simulink model "speed_pi_compare_tb"  (R2026b)
settings: Solver=FixedStepDiscrete  StopTime=0.01  FixedStep=0.0001
model workspace (MAT data in the model file):
  Iq_int_limit = 0.5
  Kaw_s = 0.08
  Ki_ASR = 1.44267798821
  Kp_ASR = 0.0180334748527
  Speed_loop_Iq_Limit = 1
  Ts = 0.0001
  Ts_ASR = 0.001
  v_ff_eps = 0.5
  v_over_eps = 3
  v_ref_zero_eps = 0
undefined symbols (not defined in the file): Iq_fric_run, Iq_fric_start, v_stick_off, v_stick_on
libraries: simulink x7

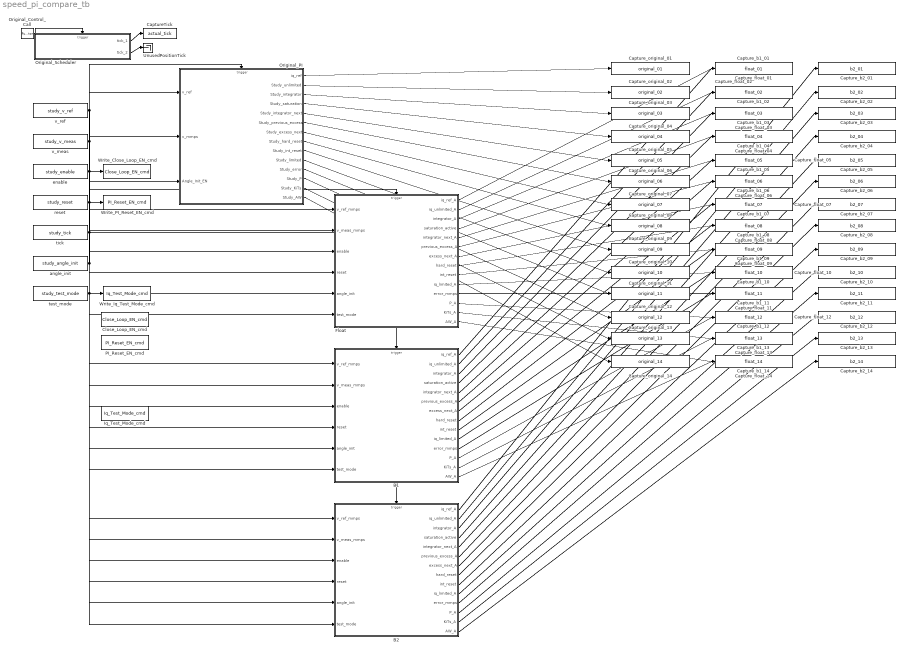
== system speed_pi_compare_tb ==
  B1 : Subsystem
  B2 : Subsystem
  CaptureTick : ToWorkspace  VariableName=actual_tick  SaveFormat=Timeseries
  Capture_b1_01 : ToWorkspace  VariableName=b1_01  SaveFormat=Timeseries
  Capture_b1_02 : ToWorkspace  VariableName=b1_02  SaveFormat=Timeseries
  Capture_b1_03 : ToWorkspace  VariableName=b1_03  SaveFormat=Timeseries
  Capture_b1_04 : ToWorkspace  VariableName=b1_04  SaveFormat=Timeseries
  Capture_b1_05 : ToWorkspace  VariableName=b1_05  SaveFormat=Timeseries
  Capture_b1_06 : ToWorkspace  VariableName=b1_06  SaveFormat=Timeseries
  Capture_b1_07 : ToWorkspace  VariableName=b1_07  SaveFormat=Timeseries
  Capture_b1_08 : ToWorkspace  VariableName=b1_08  SaveFormat=Timeseries
  Capture_b1_09 : ToWorkspace  VariableName=b1_09  SaveFormat=Timeseries
  Capture_b1_10 : ToWorkspace  VariableName=b1_10  SaveFormat=Timeseries
  Capture_b1_11 : ToWorkspace  VariableName=b1_11  SaveFormat=Timeseries
  Capture_b1_12 : ToWorkspace  VariableName=b1_12  SaveFormat=Timeseries
  Capture_b1_13 : ToWorkspace  VariableName=b1_13  SaveFormat=Timeseries
  Capture_b1_14 : ToWorkspace  VariableName=b1_14  SaveFormat=Timeseries
  Capture_b2_01 : ToWorkspace  VariableName=b2_01  SaveFormat=Timeseries
  Capture_b2_02 : ToWorkspace  VariableName=b2_02  SaveFormat=Timeseries
  Capture_b2_03 : ToWorkspace  VariableName=b2_03  SaveFormat=Timeseries
  Capture_b2_04 : ToWorkspace  VariableName=b2_04  SaveFormat=Timeseries
  Capture_b2_05 : ToWorkspace  VariableName=b2_05  SaveFormat=Timeseries
  Capture_b2_06 : ToWorkspace  VariableName=b2_06  SaveFormat=Timeseries
  Capture_b2_07 : ToWorkspace  VariableName=b2_07  SaveFormat=Timeseries
  Capture_b2_08 : ToWorkspace  VariableName=b2_08  SaveFormat=Timeseries
  Capture_b2_09 : ToWorkspace  VariableName=b2_09  SaveFormat=Timeseries
  Capture_b2_10 : ToWorkspace  VariableName=b2_10  SaveFormat=Timeseries
  Capture_b2_11 : ToWorkspace  VariableName=b2_11  SaveFormat=Timeseries
  Capture_b2_12 : ToWorkspace  VariableName=b2_12  SaveFormat=Timeseries
  Capture_b2_13 : ToWorkspace  VariableName=b2_13  SaveFormat=Timeseries
  Capture_b2_14 : ToWorkspace  VariableName=b2_14  SaveFormat=Timeseries
  Capture_float_01 : ToWorkspace  VariableName=float_01  SaveFormat=Timeseries
  Capture_float_02 : ToWorkspace  VariableName=float_02  SaveFormat=Timeseries
  Capture_float_03 : ToWorkspace  VariableName=float_03  SaveFormat=Timeseries
  Capture_float_04 : ToWorkspace  VariableName=float_04  SaveFormat=Timeseries
  Capture_float_05 : ToWorkspace  VariableName=float_05  SaveFormat=Timeseries
  Capture_float_06 : ToWorkspace  VariableName=float_06  SaveFormat=Timeseries
  Capture_float_07 : ToWorkspace  VariableName=float_07  SaveFormat=Timeseries
  Capture_float_08 : ToWorkspace  VariableName=float_08  SaveFormat=Timeseries
  Capture_float_09 : ToWorkspace  VariableName=float_09  SaveFormat=Timeseries
  Capture_float_10 : ToWorkspace  VariableName=float_10  SaveFormat=Timeseries
  Capture_float_11 : ToWorkspace  VariableName=float_11  SaveFormat=Timeseries
  Capture_float_12 : ToWorkspace  VariableName=float_12  SaveFormat=Timeseries
  Capture_float_13 : ToWorkspace  VariableName=float_13  SaveFormat=Timeseries
  Capture_float_14 : ToWorkspace  VariableName=float_14  SaveFormat=Timeseries
  Capture_original_01 : ToWorkspace  VariableName=original_01  SaveFormat=Timeseries
  Capture_original_02 : ToWorkspace  VariableName=original_02  SaveFormat=Timeseries
  Capture_original_03 : ToWorkspace  VariableName=original_03  SaveFormat=Timeseries
  Capture_original_04 : ToWorkspace  VariableName=original_04  SaveFormat=Timeseries
  Capture_original_05 : ToWorkspace  VariableName=original_05  SaveFormat=Timeseries
  Capture_original_06 : ToWorkspace  VariableName=original_06  SaveFormat=Timeseries
  Capture_original_07 : ToWorkspace  VariableName=original_07  SaveFormat=Timeseries
  Capture_original_08 : ToWorkspace  VariableName=original_08  SaveFormat=Timeseries
  Capture_original_09 : ToWorkspace  VariableName=original_09  SaveFormat=Timeseries
  Capture_original_10 : ToWorkspace  VariableName=original_10  SaveFormat=Timeseries
  Capture_original_11 : ToWorkspace  VariableName=original_11  SaveFormat=Timeseries
  Capture_original_12 : ToWorkspace  VariableName=original_12  SaveFormat=Timeseries
  Capture_original_13 : ToWorkspace  VariableName=original_13  SaveFormat=Timeseries
  Capture_original_14 : ToWorkspace  VariableName=original_14  SaveFormat=Timeseries
  Close_Loop_EN_cmd : DataStoreMemory  DataStoreName=Close_Loop_EN_cmd  ShowAdditionalParam=off
  Float : Subsystem
  Iq_Test_Mode_cmd : DataStoreMemory  DataStoreName=Iq_Test_Mode_cmd  ShowAdditionalParam=off
  Original_Control_Call : FunctionCallGenerator  SampleTime=Ts
  Original_PI : Subsystem  TreatAsAtomicUnit=on
  Original_Scheduler : Subsystem
  PI_Reset_EN_cmd : DataStoreMemory  DataStoreName=PI_Reset_EN_cmd  ShowAdditionalParam=off
  UnusedPositionTick : Terminator
  Write_Close_Loop_EN_cmd : DataStoreWrite  Priority=-10  DataStoreName=Close_Loop_EN_cmd  IndexOptions=Index vector (dialog)  Indices=1  OutputSizes=1
  Write_Iq_Test_Mode_cmd : DataStoreWrite  Priority=-10  DataStoreName=Iq_Test_Mode_cmd  IndexOptions=Index vector (dialog)  Indices=1  OutputSizes=1
  Write_PI_Reset_EN_cmd : DataStoreWrite  Priority=-10  DataStoreName=PI_Reset_EN_cmd  IndexOptions=Index vector (dialog)  Indices=1  OutputSizes=1
  angle_init : FromWorkspace  VariableName=study_angle_init  SampleTime=0.0001  Interpolate=off  OutputAfterFinalValue=Holding final value
  enable : FromWorkspace  VariableName=study_enable  SampleTime=0.0001  Interpolate=off  OutputAfterFinalValue=Holding final value
  reset : FromWorkspace  VariableName=study_reset  SampleTime=0.0001  Interpolate=off  OutputAfterFinalValue=Holding final value
  test_mode : FromWorkspace  VariableName=study_test_mode  SampleTime=0.0001  Interpolate=off  OutputAfterFinalValue=Holding final value
  tick : FromWorkspace  VariableName=study_tick  SampleTime=0.0001  Interpolate=off  OutputAfterFinalValue=Holding final value
  v_meas : FromWorkspace  VariableName=study_v_meas  SampleTime=0.0001  Interpolate=off  OutputAfterFinalValue=Holding final value
  v_ref : FromWorkspace  VariableName=study_v_ref  SampleTime=0.0001  Interpolate=off  OutputAfterFinalValue=Holding final value
  wires:
  Original_Control_Call/1 -> Original_Scheduler/Trigger
  Original_Scheduler/2(tick_2) -> UnusedPositionTick/1
  Original_Scheduler/1(tick_1) -> CaptureTick/1
  v_ref/1 -> Original_PI/1(v_ref), Float/1(v_ref_mmps), B1/1(v_ref_mmps), B2/1(v_ref_mmps)
  v_meas/1 -> Original_PI/2(v_mmps), Float/2(v_meas_mmps), B1/2(v_meas_mmps), B2/2(v_meas_mmps)
  angle_init/1 -> Original_PI/3(Angle_Init_EN), Float/5(angle_init), B1/5(angle_init), B2/5(angle_init)
  tick/1 -> Original_PI/Trigger, Float/Trigger, B1/Trigger, B2/Trigger
  enable/1 -> Write_Close_Loop_EN_cmd/1, Float/3(enable), B1/3(enable), B2/3(enable)
  reset/1 -> Write_PI_Reset_EN_cmd/1, Float/4(reset), B1/4(reset), B2/4(reset)
  test_mode/1 -> Write_Iq_Test_Mode_cmd/1, Float/6(test_mode), B1/6(test_mode), B2/6(test_mode)
  Original_PI/1(iq_ref) -> Capture_original_01/1
  Original_PI/2(Study_unlimited) -> Capture_original_02/1
  Original_PI/3(Study_integrator) -> Capture_original_03/1
  Original_PI/4(Study_saturation) -> Capture_original_04/1
  Original_PI/5(Study_integrator_next) -> Capture_original_05/1
  Original_PI/6(Study_previous_excess) -> Capture_original_06/1
  Original_PI/7(Study_excess_next) -> Capture_original_07/1
  Original_PI/8(Study_hard_reset) -> Capture_original_08/1
  Original_PI/9(Study_int_reset) -> Capture_original_09/1
  Original_PI/10(Study_limited) -> Capture_original_10/1
  Original_PI/11(Study_error) -> Capture_original_11/1
  Original_PI/12(Study_P) -> Capture_original_12/1
  Original_PI/13(Study_KiTs) -> Capture_original_13/1
  Original_PI/14(Study_AW) -> Capture_original_14/1
  Float/1(iq_ref_A) -> Capture_float_01/1
  Float/2(iq_unlimited_A) -> Capture_float_02/1
  Float/3(integrator_A) -> Capture_float_03/1
  Float/4(saturation_active) -> Capture_float_04/1
  Float/5(integrator_next_A) -> Capture_float_05/1
  Float/6(previous_excess_A) -> Capture_float_06/1
  Float/7(excess_next_A) -> Capture_float_07/1
  Float/8(hard_reset) -> Capture_float_08/1
  Float/9(int_reset) -> Capture_float_09/1
  Float/10(iq_limited_A) -> Capture_float_10/1
  Float/11(error_mmps) -> Capture_float_11/1
  Float/12(P_A) -> Capture_float_12/1
  Float/13(KiTs_A) -> Capture_float_13/1
  Float/14(AW_A) -> Capture_float_14/1
  B1/1(iq_ref_A) -> Capture_b1_01/1
  B1/2(iq_unlimited_A) -> Capture_b1_02/1
  B1/3(integrator_A) -> Capture_b1_03/1
  B1/4(saturation_active) -> Capture_b1_04/1
  B1/5(integrator_next_A) -> Capture_b1_05/1
  B1/6(previous_excess_A) -> Capture_b1_06/1
  B1/7(excess_next_A) -> Capture_b1_07/1
  B1/8(hard_reset) -> Capture_b1_08/1
  B1/9(int_reset) -> Capture_b1_09/1
  B1/10(iq_limited_A) -> Capture_b1_10/1
  B1/11(error_mmps) -> Capture_b1_11/1
  B1/12(P_A) -> Capture_b1_12/1
  B1/13(KiTs_A) -> Capture_b1_13/1
  B1/14(AW_A) -> Capture_b1_14/1
  B2/1(iq_ref_A) -> Capture_b2_01/1
  B2/2(iq_unlimited_A) -> Capture_b2_02/1
  B2/3(integrator_A) -> Capture_b2_03/1
  B2/4(saturation_active) -> Capture_b2_04/1
  B2/5(integrator_next_A) -> Capture_b2_05/1
  B2/6(previous_excess_A) -> Capture_b2_06/1
  B2/7(excess_next_A) -> Capture_b2_07/1
  B2/8(hard_reset) -> Capture_b2_08/1
  B2/9(int_reset) -> Capture_b2_09/1
  B2/10(iq_limited_A) -> Capture_b2_10/1
  B2/11(error_mmps) -> Capture_b2_11/1
  B2/12(P_A) -> Capture_b2_12/1
  B2/13(KiTs_A) -> Capture_b2_13/1
  B2/14(AW_A) -> Capture_b2_14/1

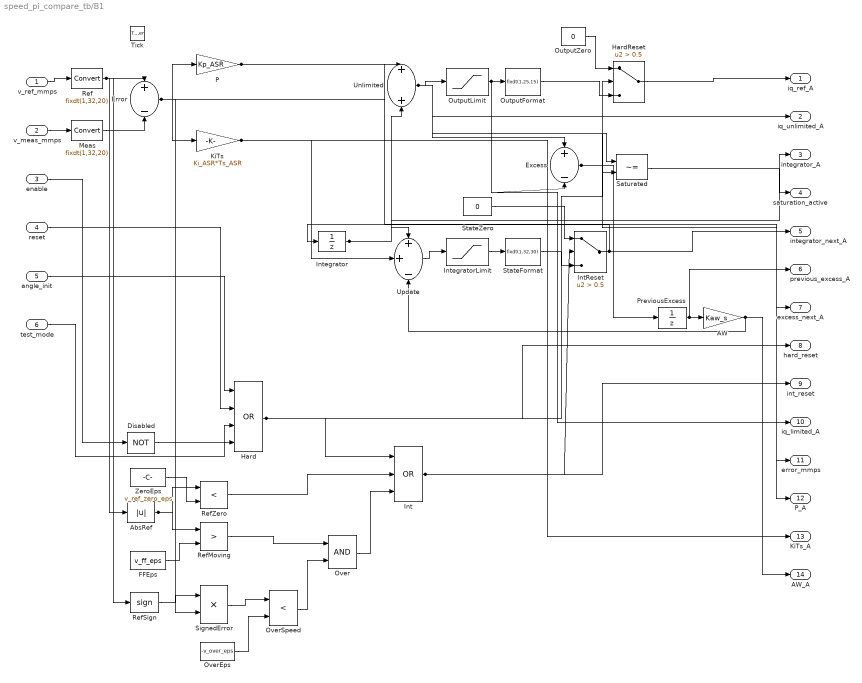
== system speed_pi_compare_tb/B1 ==
  v_ref_mmps : Inport
  v_meas_mmps : Inport  Port=2
  enable : Inport  Port=3
  reset : Inport  Port=4
  angle_init : Inport  Port=5
  test_mode : Inport  Port=6
  Tick : TriggerPort  VariantControl=(inherit)
  AW : Gain  Gain=Kaw_s  ParamDataTypeStr=fixdt(0,32,30)  OutDataTypeStr=fixdt(1,40,30)  RndMeth=Convergent  SaturateOnIntegerOverflow=on
  AbsRef : Abs  RndMeth=Convergent
  Disabled : Logic  Operator=NOT  AllPortsSameDT=off  OutDataTypeStr=boolean
  Error : Sum  Inputs=+-  OutDataTypeStr=fixdt(1,33,20)  AccumDataTypeStr=fixdt(1,33,20)  RndMeth=Convergent  SaturateOnIntegerOverflow=on
  Excess : Sum  Inputs=+-  OutDataTypeStr=fixdt(1,40,30)  AccumDataTypeStr=fixdt(1,44,30)  RndMeth=Convergent  SaturateOnIntegerOverflow=on
  FFEps : Constant  Value=v_ff_eps  OutDataTypeStr=fixdt(1,32,20)
  Hard : Logic  Operator=OR  Inputs=4  AllPortsSameDT=off  OutDataTypeStr=boolean
  HardReset : Switch  Criteria=u2 > Threshold  Threshold=0.5  RndMeth=Convergent  InputSameDT=off
  Int : Logic  Operator=OR  Inputs=3  AllPortsSameDT=off  OutDataTypeStr=boolean
  IntReset : Switch  Criteria=u2 > Threshold  Threshold=0.5  RndMeth=Convergent  InputSameDT=off
  Integrator : UnitDelay  SampleTime=-1
  IntegratorLimit : Saturate  UpperLimit=Iq_int_limit  LowerLimit=-Iq_int_limit  RndMeth=Convergent
  KiTs : Gain  Gain=Ki_ASR*Ts_ASR  ParamDataTypeStr=fixdt(0,32,30)  OutDataTypeStr=fixdt(1,40,30)  RndMeth=Convergent  SaturateOnIntegerOverflow=on
  Meas : DataTypeConversion  OutDataTypeStr=fixdt(1,32,20)  RndMeth=Convergent
  OutputFormat : DataTypeConversion  OutDataTypeStr=fixdt(1,25,15)  RndMeth=Convergent
  OutputLimit : Saturate  UpperLimit=Speed_loop_Iq_Limit  LowerLimit=-Speed_loop_Iq_Limit  RndMeth=Convergent
  OutputZero : Constant  Value=0  OutDataTypeStr=fixdt(1,25,15)
  Over : Logic  AllPortsSameDT=off  OutDataTypeStr=boolean
  OverEps : Constant  Value=-v_over_eps  OutDataTypeStr=fixdt(1,33,20)
  OverSpeed : RelationalOperator  Operator=<  RndMeth=Convergent  InputSameDT=off
  P : Gain  Gain=Kp_ASR  ParamDataTypeStr=fixdt(0,32,30)  OutDataTypeStr=fixdt(1,40,30)  RndMeth=Convergent  SaturateOnIntegerOverflow=on
  PreviousExcess : UnitDelay  SampleTime=-1
  Ref : DataTypeConversion  OutDataTypeStr=fixdt(1,32,20)  RndMeth=Convergent
  RefMoving : RelationalOperator  Operator=>  RndMeth=Convergent  InputSameDT=off
  RefSign : Signum
  RefZero : RelationalOperator  Operator=<  RndMeth=Convergent  InputSameDT=off
  Saturated : RelationalOperator  Operator=~=  RndMeth=Convergent  InputSameDT=off
  SignedError : Product  OutDataTypeStr=fixdt(1,33,20)  RndMeth=Convergent  SaturateOnIntegerOverflow=on
  StateFormat : DataTypeConversion  OutDataTypeStr=fixdt(1,32,30)  RndMeth=Convergent
  StateZero : Constant  Value=0  OutDataTypeStr=fixdt(1,32,30)
  Unlimited : Sum  OutDataTypeStr=fixdt(1,42,30)  AccumDataTypeStr=fixdt(1,44,30)  RndMeth=Convergent  SaturateOnIntegerOverflow=on
  Update : Sum  Inputs=++-  OutDataTypeStr=fixdt(1,44,30)  AccumDataTypeStr=fixdt(1,44,30)  RndMeth=Convergent  SaturateOnIntegerOverflow=on
  ZeroEps : Constant  Value=v_ref_zero_eps  OutDataTypeStr=fixdt(1,32,20)
  iq_ref_A : Outport
  iq_unlimited_A : Outport  Port=2
  integrator_A : Outport  Port=3
  saturation_active : Outport  Port=4
  integrator_next_A : Outport  Port=5
  previous_excess_A : Outport  Port=6
  excess_next_A : Outport  Port=7
  hard_reset : Outport  Port=8
  int_reset : Outport  Port=9
  iq_limited_A : Outport  Port=10
  error_mmps : Outport  Port=11
  P_A : Outport  Port=12
  KiTs_A : Outport  Port=13
  AW_A : Outport  Port=14
  wires:
  Saturated/1 -> saturation_active/1
  HardReset/1 -> iq_ref_A/1
  Over/1 -> Int/3
  RefZero/1 -> Int/2
  OverSpeed/1 -> Over/2
  RefMoving/1 -> Over/1
  OverEps/1 -> OverSpeed/2
  SignedError/1 -> OverSpeed/1
  RefSign/1 -> SignedError/1
  FFEps/1 -> RefMoving/2
  ZeroEps/1 -> RefZero/2
  AbsRef/1 -> RefMoving/1, RefZero/1
  Disabled/1 -> Hard/4
  test_mode/1 -> Hard/3
  reset/1 -> Hard/2
  angle_init/1 -> Hard/1
  enable/1 -> Disabled/1
  OutputFormat/1 -> HardReset/3
  Hard/1 -> hard_reset/1, Int/1, HardReset/2
  OutputZero/1 -> HardReset/1
  IntReset/1 -> integrator_next_A/1, Integrator/1
  StateFormat/1 -> IntReset/3
  Int/1 -> int_reset/1, IntReset/2
  StateZero/1 -> IntReset/1
  IntegratorLimit/1 -> StateFormat/1
  Update/1 -> IntegratorLimit/1
  AW/1 -> AW_A/1, Update/3
  KiTs/1 -> KiTs_A/1, Update/2
  PreviousExcess/1 -> previous_excess_A/1, AW/1
  Excess/1 -> excess_next_A/1, PreviousExcess/1
  OutputLimit/1 -> iq_limited_A/1, Saturated/2, Excess/2, OutputFormat/1
  Unlimited/1 -> iq_unlimited_A/1, Saturated/1, Excess/1, OutputLimit/1
  Integrator/1 -> integrator_A/1, Update/1, Unlimited/2
  P/1 -> P_A/1, Unlimited/1
  Error/1 -> error_mmps/1, SignedError/2, KiTs/1, P/1
  Meas/1 -> Error/2
  Ref/1 -> RefSign/1, AbsRef/1, Error/1
  v_meas_mmps/1 -> Meas/1
  v_ref_mmps/1 -> Ref/1

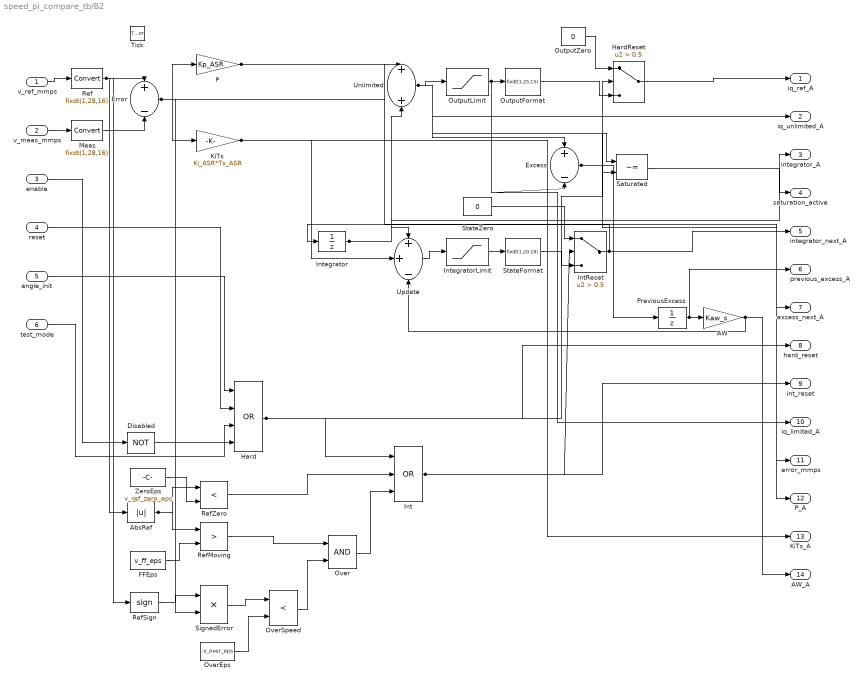
== system speed_pi_compare_tb/B2 ==
  v_ref_mmps : Inport
  v_meas_mmps : Inport  Port=2
  enable : Inport  Port=3
  reset : Inport  Port=4
  angle_init : Inport  Port=5
  test_mode : Inport  Port=6
  Tick : TriggerPort  VariantControl=(inherit)
  AW : Gain  Gain=Kaw_s  ParamDataTypeStr=fixdt(0,24,22)  OutDataTypeStr=fixdt(1,28,18)  RndMeth=Convergent  SaturateOnIntegerOverflow=on
  AbsRef : Abs  RndMeth=Convergent
  Disabled : Logic  Operator=NOT  AllPortsSameDT=off  OutDataTypeStr=boolean
  Error : Sum  Inputs=+-  OutDataTypeStr=fixdt(1,29,16)  AccumDataTypeStr=fixdt(1,29,16)  RndMeth=Convergent  SaturateOnIntegerOverflow=on
  Excess : Sum  Inputs=+-  OutDataTypeStr=fixdt(1,28,18)  AccumDataTypeStr=fixdt(1,32,18)  RndMeth=Convergent  SaturateOnIntegerOverflow=on
  FFEps : Constant  Value=v_ff_eps  OutDataTypeStr=fixdt(1,28,16)
  Hard : Logic  Operator=OR  Inputs=4  AllPortsSameDT=off  OutDataTypeStr=boolean
  HardReset : Switch  Criteria=u2 > Threshold  Threshold=0.5  RndMeth=Convergent  InputSameDT=off
  Int : Logic  Operator=OR  Inputs=3  AllPortsSameDT=off  OutDataTypeStr=boolean
  IntReset : Switch  Criteria=u2 > Threshold  Threshold=0.5  RndMeth=Convergent  InputSameDT=off
  Integrator : UnitDelay  SampleTime=-1
  IntegratorLimit : Saturate  UpperLimit=Iq_int_limit  LowerLimit=-Iq_int_limit  RndMeth=Convergent
  KiTs : Gain  Gain=Ki_ASR*Ts_ASR  ParamDataTypeStr=fixdt(0,24,22)  OutDataTypeStr=fixdt(1,28,18)  RndMeth=Convergent  SaturateOnIntegerOverflow=on
  Meas : DataTypeConversion  OutDataTypeStr=fixdt(1,28,16)  RndMeth=Convergent
  OutputFormat : DataTypeConversion  OutDataTypeStr=fixdt(1,25,15)  RndMeth=Convergent
  OutputLimit : Saturate  UpperLimit=Speed_loop_Iq_Limit  LowerLimit=-Speed_loop_Iq_Limit  RndMeth=Convergent
  OutputZero : Constant  Value=0  OutDataTypeStr=fixdt(1,25,15)
  Over : Logic  AllPortsSameDT=off  OutDataTypeStr=boolean
  OverEps : Constant  Value=-v_over_eps  OutDataTypeStr=fixdt(1,29,16)
  OverSpeed : RelationalOperator  Operator=<  RndMeth=Convergent  InputSameDT=off
  P : Gain  Gain=Kp_ASR  ParamDataTypeStr=fixdt(0,24,22)  OutDataTypeStr=fixdt(1,28,18)  RndMeth=Convergent  SaturateOnIntegerOverflow=on
  PreviousExcess : UnitDelay  SampleTime=-1
  Ref : DataTypeConversion  OutDataTypeStr=fixdt(1,28,16)  RndMeth=Convergent
  RefMoving : RelationalOperator  Operator=>  RndMeth=Convergent  InputSameDT=off
  RefSign : Signum
  RefZero : RelationalOperator  Operator=<  RndMeth=Convergent  InputSameDT=off
  Saturated : RelationalOperator  Operator=~=  RndMeth=Convergent  InputSameDT=off
  SignedError : Product  OutDataTypeStr=fixdt(1,29,16)  RndMeth=Convergent  SaturateOnIntegerOverflow=on
  StateFormat : DataTypeConversion  OutDataTypeStr=fixdt(1,20,18)  RndMeth=Convergent
  StateZero : Constant  Value=0  OutDataTypeStr=fixdt(1,20,18)
  Unlimited : Sum  OutDataTypeStr=fixdt(1,30,18)  AccumDataTypeStr=fixdt(1,32,18)  RndMeth=Convergent  SaturateOnIntegerOverflow=on
  Update : Sum  Inputs=++-  OutDataTypeStr=fixdt(1,32,18)  AccumDataTypeStr=fixdt(1,32,18)  RndMeth=Convergent  SaturateOnIntegerOverflow=on
  ZeroEps : Constant  Value=v_ref_zero_eps  OutDataTypeStr=fixdt(1,28,16)
  iq_ref_A : Outport
  iq_unlimited_A : Outport  Port=2
  integrator_A : Outport  Port=3
  saturation_active : Outport  Port=4
  integrator_next_A : Outport  Port=5
  previous_excess_A : Outport  Port=6
  excess_next_A : Outport  Port=7
  hard_reset : Outport  Port=8
  int_reset : Outport  Port=9
  iq_limited_A : Outport  Port=10
  error_mmps : Outport  Port=11
  P_A : Outport  Port=12
  KiTs_A : Outport  Port=13
  AW_A : Outport  Port=14
  wires:
  Saturated/1 -> saturation_active/1
  HardReset/1 -> iq_ref_A/1
  Over/1 -> Int/3
  RefZero/1 -> Int/2
  OverSpeed/1 -> Over/2
  RefMoving/1 -> Over/1
  OverEps/1 -> OverSpeed/2
  SignedError/1 -> OverSpeed/1
  RefSign/1 -> SignedError/1
  FFEps/1 -> RefMoving/2
  ZeroEps/1 -> RefZero/2
  AbsRef/1 -> RefMoving/1, RefZero/1
  Disabled/1 -> Hard/4
  test_mode/1 -> Hard/3
  reset/1 -> Hard/2
  angle_init/1 -> Hard/1
  enable/1 -> Disabled/1
  OutputFormat/1 -> HardReset/3
  Hard/1 -> hard_reset/1, Int/1, HardReset/2
  OutputZero/1 -> HardReset/1
  IntReset/1 -> integrator_next_A/1, Integrator/1
  StateFormat/1 -> IntReset/3
  Int/1 -> int_reset/1, IntReset/2
  StateZero/1 -> IntReset/1
  IntegratorLimit/1 -> StateFormat/1
  Update/1 -> IntegratorLimit/1
  AW/1 -> AW_A/1, Update/3
  KiTs/1 -> KiTs_A/1, Update/2
  PreviousExcess/1 -> previous_excess_A/1, AW/1
  Excess/1 -> excess_next_A/1, PreviousExcess/1
  OutputLimit/1 -> iq_limited_A/1, Saturated/2, Excess/2, OutputFormat/1
  Unlimited/1 -> iq_unlimited_A/1, Saturated/1, Excess/1, OutputLimit/1
  Integrator/1 -> integrator_A/1, Update/1, Unlimited/2
  P/1 -> P_A/1, Unlimited/1
  Error/1 -> error_mmps/1, SignedError/2, KiTs/1, P/1
  Meas/1 -> Error/2
  Ref/1 -> RefSign/1, AbsRef/1, Error/1
  v_meas_mmps/1 -> Meas/1
  v_ref_mmps/1 -> Ref/1

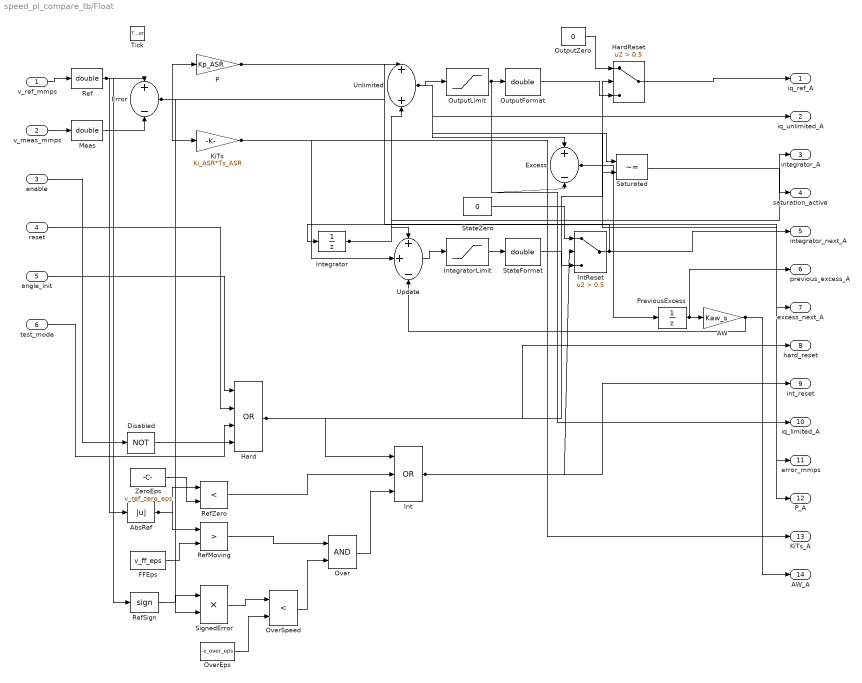
== system speed_pi_compare_tb/Float ==
  v_ref_mmps : Inport
  v_meas_mmps : Inport  Port=2
  enable : Inport  Port=3
  reset : Inport  Port=4
  angle_init : Inport  Port=5
  test_mode : Inport  Port=6
  Tick : TriggerPort  VariantControl=(inherit)
  AW : Gain  Gain=Kaw_s  ParamDataTypeStr=double  OutDataTypeStr=double  RndMeth=Convergent  SaturateOnIntegerOverflow=on
  AbsRef : Abs  RndMeth=Convergent
  Disabled : Logic  Operator=NOT  AllPortsSameDT=off  OutDataTypeStr=boolean
  Error : Sum  Inputs=+-  OutDataTypeStr=double  AccumDataTypeStr=double  RndMeth=Convergent  SaturateOnIntegerOverflow=on
  Excess : Sum  Inputs=+-  OutDataTypeStr=double  AccumDataTypeStr=double  RndMeth=Convergent  SaturateOnIntegerOverflow=on
  FFEps : Constant  Value=v_ff_eps  OutDataTypeStr=double
  Hard : Logic  Operator=OR  Inputs=4  AllPortsSameDT=off  OutDataTypeStr=boolean
  HardReset : Switch  Criteria=u2 > Threshold  Threshold=0.5  RndMeth=Convergent  InputSameDT=off
  Int : Logic  Operator=OR  Inputs=3  AllPortsSameDT=off  OutDataTypeStr=boolean
  IntReset : Switch  Criteria=u2 > Threshold  Threshold=0.5  RndMeth=Convergent  InputSameDT=off
  Integrator : UnitDelay  SampleTime=-1
  IntegratorLimit : Saturate  UpperLimit=Iq_int_limit  LowerLimit=-Iq_int_limit  RndMeth=Convergent
  KiTs : Gain  Gain=Ki_ASR*Ts_ASR  ParamDataTypeStr=double  OutDataTypeStr=double  RndMeth=Convergent  SaturateOnIntegerOverflow=on
  Meas : DataTypeConversion  OutDataTypeStr=double  RndMeth=Convergent
  OutputFormat : DataTypeConversion  OutDataTypeStr=double  RndMeth=Convergent
  OutputLimit : Saturate  UpperLimit=Speed_loop_Iq_Limit  LowerLimit=-Speed_loop_Iq_Limit  RndMeth=Convergent
  OutputZero : Constant  Value=0  OutDataTypeStr=double
  Over : Logic  AllPortsSameDT=off  OutDataTypeStr=boolean
  OverEps : Constant  Value=-v_over_eps  OutDataTypeStr=double
  OverSpeed : RelationalOperator  Operator=<  RndMeth=Convergent  InputSameDT=off
  P : Gain  Gain=Kp_ASR  ParamDataTypeStr=double  OutDataTypeStr=double  RndMeth=Convergent  SaturateOnIntegerOverflow=on
  PreviousExcess : UnitDelay  SampleTime=-1
  Ref : DataTypeConversion  OutDataTypeStr=double  RndMeth=Convergent
  RefMoving : RelationalOperator  Operator=>  RndMeth=Convergent  InputSameDT=off
  RefSign : Signum
  RefZero : RelationalOperator  Operator=<  RndMeth=Convergent  InputSameDT=off
  Saturated : RelationalOperator  Operator=~=  RndMeth=Convergent  InputSameDT=off
  SignedError : Product  OutDataTypeStr=double  RndMeth=Convergent  SaturateOnIntegerOverflow=on
  StateFormat : DataTypeConversion  OutDataTypeStr=double  RndMeth=Convergent
  StateZero : Constant  Value=0  OutDataTypeStr=double
  Unlimited : Sum  OutDataTypeStr=double  AccumDataTypeStr=double  RndMeth=Convergent  SaturateOnIntegerOverflow=on
  Update : Sum  Inputs=++-  OutDataTypeStr=double  AccumDataTypeStr=double  RndMeth=Convergent  SaturateOnIntegerOverflow=on
  ZeroEps : Constant  Value=v_ref_zero_eps  OutDataTypeStr=double
  iq_ref_A : Outport
  iq_unlimited_A : Outport  Port=2
  integrator_A : Outport  Port=3
  saturation_active : Outport  Port=4
  integrator_next_A : Outport  Port=5
  previous_excess_A : Outport  Port=6
  excess_next_A : Outport  Port=7
  hard_reset : Outport  Port=8
  int_reset : Outport  Port=9
  iq_limited_A : Outport  Port=10
  error_mmps : Outport  Port=11
  P_A : Outport  Port=12
  KiTs_A : Outport  Port=13
  AW_A : Outport  Port=14
  wires:
  Saturated/1 -> saturation_active/1
  HardReset/1 -> iq_ref_A/1
  Over/1 -> Int/3
  RefZero/1 -> Int/2
  OverSpeed/1 -> Over/2
  RefMoving/1 -> Over/1
  OverEps/1 -> OverSpeed/2
  SignedError/1 -> OverSpeed/1
  RefSign/1 -> SignedError/1
  FFEps/1 -> RefMoving/2
  ZeroEps/1 -> RefZero/2
  AbsRef/1 -> RefMoving/1, RefZero/1
  Disabled/1 -> Hard/4
  test_mode/1 -> Hard/3
  reset/1 -> Hard/2
  angle_init/1 -> Hard/1
  enable/1 -> Disabled/1
  OutputFormat/1 -> HardReset/3
  Hard/1 -> hard_reset/1, Int/1, HardReset/2
  OutputZero/1 -> HardReset/1
  IntReset/1 -> integrator_next_A/1, Integrator/1
  StateFormat/1 -> IntReset/3
  Int/1 -> int_reset/1, IntReset/2
  StateZero/1 -> IntReset/1
  IntegratorLimit/1 -> StateFormat/1
  Update/1 -> IntegratorLimit/1
  AW/1 -> AW_A/1, Update/3
  KiTs/1 -> KiTs_A/1, Update/2
  PreviousExcess/1 -> previous_excess_A/1, AW/1
  Excess/1 -> excess_next_A/1, PreviousExcess/1
  OutputLimit/1 -> iq_limited_A/1, Saturated/2, Excess/2, OutputFormat/1
  Unlimited/1 -> iq_unlimited_A/1, Saturated/1, Excess/1, OutputLimit/1
  Integrator/1 -> integrator_A/1, Update/1, Unlimited/2
  P/1 -> P_A/1, Unlimited/1
  Error/1 -> error_mmps/1, SignedError/2, KiTs/1, P/1
  Meas/1 -> Error/2
  Ref/1 -> RefSign/1, AbsRef/1, Error/1
  v_meas_mmps/1 -> Meas/1
  v_ref_mmps/1 -> Ref/1

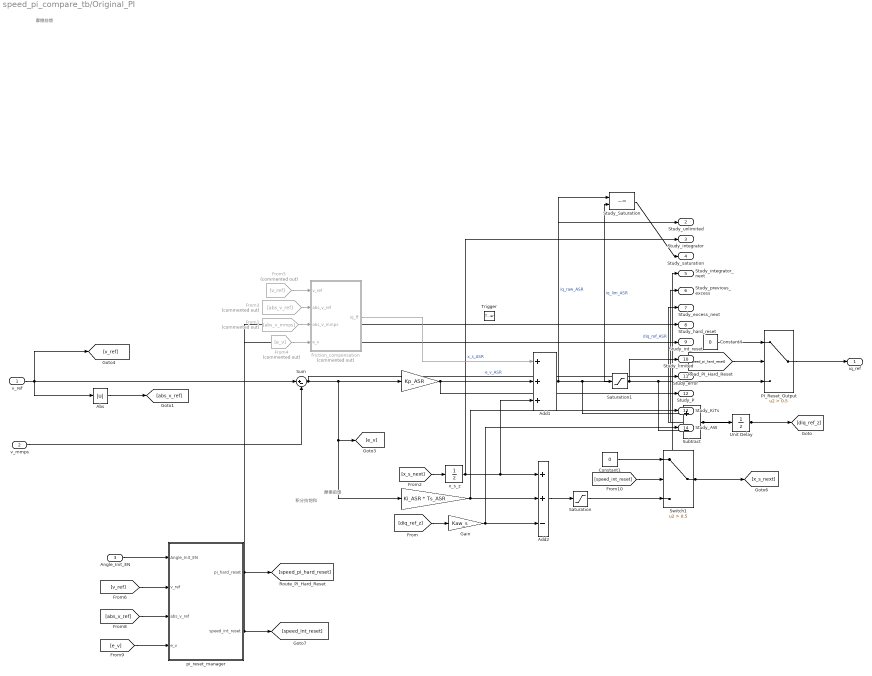
== system speed_pi_compare_tb/Original_PI ==
  note: 摩擦前馈
  note: 积分抗饱和
  note: 摩擦前馈
  v_ref : Inport
  v_mmps : Inport  Port=2
  Angle_Init_EN : Inport  Port=3
  Trigger : TriggerPort  VariantControl=(inherit)
  " " : Gain  Gain=Ki_ASR * Ts_ASR
  "  " : Gain  Gain=Kp_ASR
  Abs : Abs  SaturateOnIntegerOverflow=off
  Add1 : Sum  Inputs=+++
  Add2 : Sum  Inputs=++-
  Constant1 : Constant  Value=0
  Constant4 : Constant  Value=0
  From1 : From  Commented=on  GotoTag=abs_v_mmps
  From3 : From  Commented=on  GotoTag=abs_v_ref
  From4 : From  Commented=on  GotoTag=e_v
  From5 : From  Commented=on  GotoTag=v_ref
  Gain : Gain  Gain=Kaw_s
  PI_Reset_Output : Switch  Criteria=u2 > Threshold  Threshold=0.5  SaturateOnIntegerOverflow=off  InputSameDT=off
  Saturation : Saturate  UpperLimit=Iq_int_limit  LowerLimit=-Iq_int_limit
  Saturation1 : Saturate  UpperLimit=Speed_loop_Iq_Limit  LowerLimit=-Speed_loop_Iq_Limit
  Study_Saturation : RelationalOperator  Operator=~=
  Subtract : Sum  Inputs=+-
  Sum : Sum  Inputs=|+-
  Switch1 : Switch  Criteria=u2 > Threshold  Threshold=0.5  SaturateOnIntegerOverflow=off  InputSameDT=off
  Unit Delay : UnitDelay  SampleTime=-1
  friction_compensation : Subsystem  Commented=on
  pi_reset_manager : Subsystem
  x_s_z : UnitDelay  SampleTime=-1
  iq_ref : Outport
  Study_unlimited : Outport  Port=2
  Study_integrator : Outport  Port=3
  Study_saturation : Outport  Port=4
  Study_integrator_next : Outport  Port=5
  Study_previous_excess : Outport  Port=6
  Study_excess_next : Outport  Port=7
  Study_hard_reset : Outport  Port=8
  Study_int_reset : Outport  Port=9
  Study_limited : Outport  Port=10
  Study_error : Outport  Port=11
  Study_P : Outport  Port=12
  Study_KiTs : Outport  Port=13
  Study_AW : Outport  Port=14
  wires:
  v_mmps/1 -> Sum/2
  Saturation/1 -> Switch1/3
  Switch1/1 -> [x_s_next], Study_integrator_next/1
  [speed_int_reset] -> Switch1/2
  pi_reset_manager/1(pi_hard_reset) -> [speed_pi_hard_reset], Study_hard_reset/1
  pi_reset_manager/2(speed_int_reset) -> [speed_int_reset], Study_int_reset/1
  [speed_pi_hard_reset] -> PI_Reset_Output/2
  [e_v] -> pi_reset_manager/4(e_v)
  [abs_v_ref] -> pi_reset_manager/3(abs_v_ref)
  [v_ref] -> pi_reset_manager/2(v_ref)
  From5/1 -> friction_compensation/1(v_ref)
  Angle_Init_EN/1 -> pi_reset_manager/1(Angle_Init_EN)
  Abs/1 -> [abs_v_ref]
  From3/1 -> friction_compensation/2(abs_v_ref)
  From1/1 -> friction_compensation/3(abs_v_mmps)
  From4/1 -> friction_compensation/4(e_v)
  x_s_z/1 -> Add2/1, Add1/3, Study_integrator/1  "x_s_ASR"
  friction_compensation/1(iq_ff) -> Add1/1
  "  "/1 -> Add1/2, Study_P/1
  Constant4/1 -> PI_Reset_Output/1
  PI_Reset_Output/1 -> iq_ref/1
  Constant1/1 -> Switch1/1
  [diq_ref_z] -> Gain/1
  Unit Delay/1 -> [diq_ref_z], Study_previous_excess/1
  Subtract/1 -> Unit Delay/1, Study_excess_next/1  "diq_ref_ASR"
  " "/1 -> Add2/2, Study_KiTs/1
  Gain/1 -> Add2/3, Study_AW/1
  Add2/1 -> Saturation/1
  [x_s_next] -> x_s_z/1
  Saturation1/1 -> Subtract/2, PI_Reset_Output/3, Study_limited/1, Study_Saturation/2  "iq_lim_ASR"
  v_ref/1 -> [v_ref], Abs/1, Sum/1
  Add1/1 -> Saturation1/1, Subtract/1, Study_unlimited/1, Study_Saturation/1  "iq_raw_ASR"
  Sum/1 -> "  "/1, " "/1, [e_v], Study_error/1  "e_v_ASR"
  Study_Saturation/1 -> Study_saturation/1

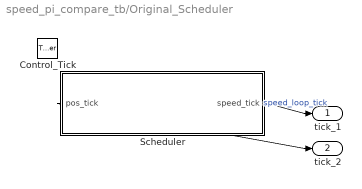
== system speed_pi_compare_tb/Original_Scheduler ==
  Control_Tick : TriggerPort  TriggerType=function-call  VariantControl=(inherit)
  Scheduler : Subsystem
  tick_1 : Outport
  tick_2 : Outport  Port=2
  wires:
  Scheduler/1(speed_tick) -> tick_1/1  "speed_loop_tick"
  Scheduler/2(pos_tick) -> tick_2/1

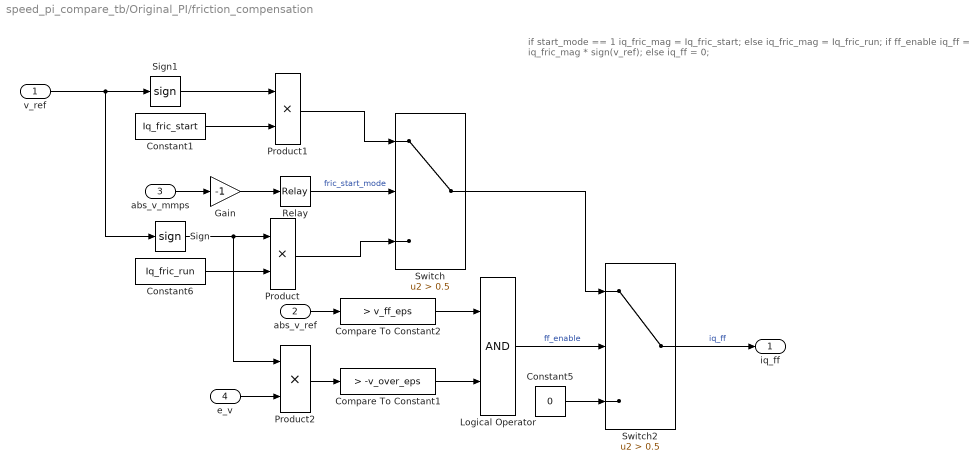
== system speed_pi_compare_tb/Original_PI/friction_compensation ==
  note: if start_mode == 1
      | 	iq_fric_mag = Iq_fric_start;
      | else
      | 	iq_fric_mag = Iq_fric_run;
      |
      | if ff_enable
      | 	iq_ff = iq_fric_mag * sign(v_ref);
      |  else
      | 	iq_ff = 0;
  v_ref : Inport
  abs_v_ref : Inport  Port=2
  abs_v_mmps : Inport  Port=3
  e_v : Inport  Port=4
  Compare To Constant1 : simulink/Logic and Bit Operations/Compare To Constant  relop=>  const=-v_over_eps  OutDataTypeStr=boolean
  Compare To Constant2 : simulink/Logic and Bit Operations/Compare To Constant  relop=>  const=v_ff_eps  OutDataTypeStr=boolean
  Constant1 : Constant  Value=Iq_fric_start
  Constant5 : Constant  Value=0
  Constant6 : Constant  Value=Iq_fric_run
  Gain : Gain  Gain=-1
  Logical Operator : Logic  AllPortsSameDT=off  OutDataTypeStr=boolean
  Product : Product
  Product1 : Product
  Product2 : Product
  Relay : Relay  OnSwitchValue=-v_stick_on  OffSwitchValue=-v_stick_off
  Sign : Signum
  Sign1 : Signum
  Switch : Switch  Criteria=u2 > Threshold  Threshold=0.5  SaturateOnIntegerOverflow=off  InputSameDT=off
  Switch2 : Switch  Criteria=u2 > Threshold  Threshold=0.5  SaturateOnIntegerOverflow=off  InputSameDT=off
  iq_ff : Outport
  wires:
  Gain/1 -> Relay/1
  Relay/1 -> Switch/2  "fric_start_mode"
  abs_v_mmps/1 -> Gain/1
  Logical Operator/1 -> Switch2/2  "ff_enable"
  Compare To Constant1/1 -> Logical Operator/2
  Compare To Constant2/1 -> Logical Operator/1
  Product2/1 -> Compare To Constant1/1
  e_v/1 -> Product2/2
  Product1/1 -> Switch/1
  Constant1/1 -> Product1/2
  Sign1/1 -> Product1/1
  Product/1 -> Switch/3
  Switch/1 -> Switch2/1
  Switch2/1 -> iq_ff/1  "iq_ff"
  abs_v_ref/1 -> Compare To Constant2/1
  Constant6/1 -> Product/2
  Constant5/1 -> Switch2/3
  Sign/1 -> Product/1, Product2/1
  v_ref/1 -> Sign1/1, Sign/1

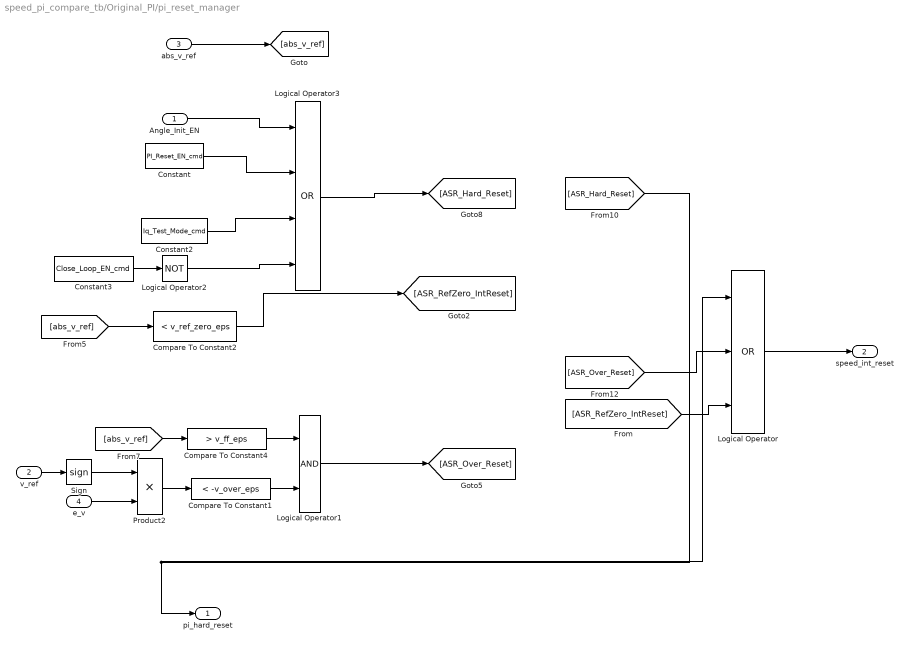
== system speed_pi_compare_tb/Original_PI/pi_reset_manager ==
  Angle_Init_EN : Inport
  v_ref : Inport  Port=2
  abs_v_ref : Inport  Port=3
  e_v : Inport  Port=4
  Compare To Constant1 : simulink/Logic and Bit Operations/Compare To Constant  relop=<  const=-v_over_eps  OutDataTypeStr=boolean
  Compare To Constant2 : simulink/Logic and Bit Operations/Compare To Constant  relop=<  const=v_ref_zero_eps  OutDataTypeStr=boolean
  Compare To Constant4 : simulink/Logic and Bit Operations/Compare To Constant  relop=>  const=v_ff_eps  OutDataTypeStr=boolean
  Constant : DataStoreRead  DataStoreName=PI_Reset_EN_cmd  IndexOptions=Index vector (dialog)  Indices=1  OutputSizes=1
  Constant2 : DataStoreRead  DataStoreName=Iq_Test_Mode_cmd  IndexOptions=Index vector (dialog)  Indices=1  OutputSizes=1
  Constant3 : DataStoreRead  DataStoreName=Close_Loop_EN_cmd  IndexOptions=Index vector (dialog)  Indices=1  OutputSizes=1
  Logical Operator : Logic  Operator=OR  Inputs=3  AllPortsSameDT=off  OutDataTypeStr=boolean
  Logical Operator1 : Logic  AllPortsSameDT=off  OutDataTypeStr=boolean
  Logical Operator2 : Logic  Operator=NOT  AllPortsSameDT=off  OutDataTypeStr=boolean
  Logical Operator3 : Logic  Operator=OR  Inputs=4  AllPortsSameDT=off  OutDataTypeStr=boolean
  Product2 : Product
  Sign : Signum
  pi_hard_reset : Outport
  speed_int_reset : Outport  Port=2
  wires:
  Constant/1 -> Logical Operator3/2
  Constant3/1 -> Logical Operator2/1
  Constant2/1 -> Logical Operator3/3
  Logical Operator2/1 -> Logical Operator3/4
  Angle_Init_EN/1 -> Logical Operator3/1
  Logical Operator3/1 -> [ASR_Hard_Reset]
  [ASR_Hard_Reset] -> Logical Operator/1, pi_hard_reset/1
  [ASR_Over_Reset] -> Logical Operator/2
  Logical Operator/1 -> speed_int_reset/1
  [ASR_RefZero_IntReset] -> Logical Operator/3
  Logical Operator1/1 -> [ASR_Over_Reset]
  abs_v_ref/1 -> [abs_v_ref]
  v_ref/1 -> Sign/1
  Compare To Constant4/1 -> Logical Operator1/1
  Compare To Constant1/1 -> Logical Operator1/2
  Product2/1 -> Compare To Constant1/1
  Sign/1 -> Product2/1
  e_v/1 -> Product2/2
  [abs_v_ref] -> Compare To Constant4/1
  [abs_v_ref] -> Compare To Constant2/1
  Compare To Constant2/1 -> [ASR_RefZero_IntReset]

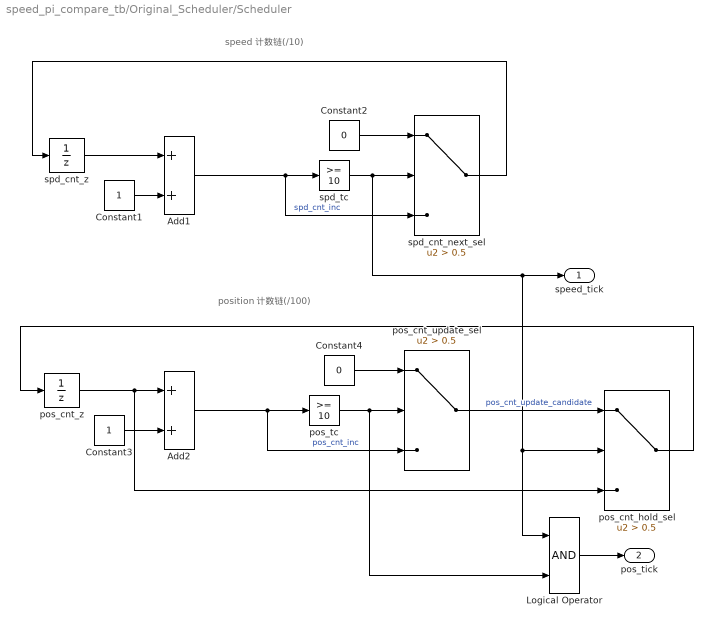
== system speed_pi_compare_tb/Original_Scheduler/Scheduler ==
  note: speed 计数链(/10)
  note: position 计数链(/100)
  Add1 : Sum
  Add2 : Sum
  Constant1 : Constant
  Constant2 : Constant  Value=0
  Constant3 : Constant
  Constant4 : Constant  Value=0
  Logical Operator : Logic  AllPortsSameDT=off  OutDataTypeStr=boolean
  pos_cnt_hold_sel : Switch  Criteria=u2 > Threshold  Threshold=0.5  SaturateOnIntegerOverflow=off  InputSameDT=off
  pos_cnt_update_sel : Switch  Criteria=u2 > Threshold  Threshold=0.5  SaturateOnIntegerOverflow=off  InputSameDT=off
  pos_cnt_z : UnitDelay  SampleTime=-1
  pos_tc : simulink/Logic and Bit Operations/Compare To Constant  relop=>=  const=10  OutDataTypeStr=boolean
  spd_cnt_next_sel : Switch  Criteria=u2 > Threshold  Threshold=0.5  SaturateOnIntegerOverflow=off  InputSameDT=off
  spd_cnt_z : UnitDelay  SampleTime=-1
  spd_tc : simulink/Logic and Bit Operations/Compare To Constant  relop=>=  const=10  OutDataTypeStr=boolean
  speed_tick : Outport
  pos_tick : Outport  Port=2
  wires:
  Logical Operator/1 -> pos_tick/1
  pos_cnt_hold_sel/1 -> pos_cnt_z/1
  pos_cnt_update_sel/1 -> pos_cnt_hold_sel/1  "pos_cnt_update_candidate"
  Constant4/1 -> pos_cnt_update_sel/1
  pos_tc/1 -> pos_cnt_update_sel/2, Logical Operator/2
  Add2/1 -> pos_tc/1, pos_cnt_update_sel/3  "pos_cnt_inc"
  Constant3/1 -> Add2/2
  pos_cnt_z/1 -> pos_cnt_hold_sel/3, Add2/1
  Add1/1 -> spd_tc/1, spd_cnt_next_sel/3  "spd_cnt_inc"
  spd_cnt_next_sel/1 -> spd_cnt_z/1
  Constant2/1 -> spd_cnt_next_sel/1
  Constant1/1 -> Add1/2
  spd_tc/1 -> spd_cnt_next_sel/2, pos_cnt_hold_sel/2, Logical Operator/1, speed_tick/1
  spd_cnt_z/1 -> Add1/1
